simulink model "Torque_Vectoring_Controller_Boon"  (R2016a)
settings: Solver=ode45  StartTime=0.0  StopTime=inf  RelTol=1e-3
InitFcn:
  | clear_close
  | dataCar
  | optParam
  | structSensors
  | structSettings
  | structEstimPar
  | structAero
  | structVariables
  | readFuzzyFile
StartFcn:
  | clear_close
  | dataCar
  | optParam
  | structSensors
  | structSettings
  | structEstimPar
  | structAero
  | structVariables
  | readFuzzyFile
values from neighbouring files (symbols this model uses):
  mu = [0.05;0.05;0.05;0.05]    [frictionfrank.m]
undefined symbols (not defined in the file or in its folder): car, optPar, tire_radius
libraries: CarMaker4SL x42, simulink x11, fuzblock x1
(part 3 of 3)

== matlab function Torque_Vectoring_Controller_Boon/CarMaker/Controls/Control Systems/Traction Control ==
  data: sensors input; Torques output; settings input; estimPar input; torqueDistribution input; slipSet input; car parameter; TiTi2 output; error output
function [Torques, TiTi2, error] = Traction(sensors, settings, estimPar, torqueDistribution, slipSet, car)

error =[0 0 0 0]';
persistent errorInt; if isempty(errorInt); errorInt=[0 0 0 0]'; end
persistent errorD; if isempty(errorD); errorD=[0 0 0 0]'; end
persistent errorPrev; if isempty(errorPrev); errorPrev=[0 0 0 0]'; end

%persistent wi_prev; if isempty(wi_prev); wi_prev=[0 0 0 0]'; end
%persistent SR_expected; if isempty(SR_expected); SR_expected=zeros(4, 8); end
%persistent wvi_prev; if isempty(wvi_prev); wvi_prev=[0 0 0 0]'; end

persistent TiPrev; if isempty(TiPrev); TiPrev=[0 0 0 0]'; end

persistent errorInt2; if isempty(errorInt2); errorInt2=[0 0 0 0]'; end
persistent Ti; if isempty(Ti); Ti=[0 0 0 0]'; end
persistent Ti2; if isempty(Ti2); Ti2=[0 0 0 0]'; end


if settings.TC == 1

    slipRatioTarget = slipSet;
    dist = estimPar.Fzi/sum(estimPar.Fzi);
    
    Kp = 100*dist*10;
    Ki = 40*dist*1000;
    Kd = 0*dist/100;
    Kv = 70/100;
    Mu = 140;
    
    Kp2 = 20*dist/1000;
    Ki2 = 40*dist/1000;
    
    %normal non linear torque control
    error = slipRatioTarget - estimPar.slip;
    
    errorInt = errorInt + error*car.dt;
    errorInt = min(max(errorInt,-0.001*[1;1;1;1]),0.003*[1;1;1;1]);
    errorD = min(max(errorD*0.1 + 0.9*(error - errorPrev)/car.dt,-25),25);
    lambdaD = Kp.*error + Ki.*errorInt + Kd.*errorD;
    Ti = lambdaD*car.tireInertia*max(estimPar.v,0)^Kv/car.tireRadius + sign(torqueDistribution).*estimPar.Fzi*(Mu/100)*car.tireRadius;
    Ti = Ti / car.gearRatio;
    
    %optimum seeking
    dFds = dFdsCalculator(estimPar.Fxi,estimPar.slip);
    error2 = dFds - 0;
    errorInt2 = errorInt2 + error2*car.dt;
    errorInt2 = min(max(errorInt2,-500*[1;1;1;1]),500*[1;1;1;1]);
    lambdaD2 = Kp2.*error2 + Ki2.*errorInt2;
    Ti2 = lambdaD2*car.tireInertia*max(estimPar.v,0)^Kv/car.tireRadius + sign(torqueDistribution).*estimPar.Fzi*(car.TC_mu)*car.tireRadius;
    Ti2 = Ti2 / car.gearRatio;
    
%     for i=1:4
%         if abs(error(i)) < 0.05
%             Ti(i) = Ti2(i);
%         end
%     end
    
    if estimPar.v < 1/3.6
        %Ti = [80 80 180 180]';
        errorInt = [0 0 0 0]';
    end

    if sensors.throttle < 0.1
        errorInt = [0 0 0 0]';
    end
    
    lowerBoundary = TiPrev - 100/car.gearRatio;
    upperBoundary = TiPrev + 100/car.gearRatio;

    Ti = min(max(Ti,lowerBoundary),upperBoundary);
    
    TiPrev = Ti;
    errorPrev = error;
    
    Torques = Ti;
    for i=1:4
        if torqueDistribution(i) > 0
            Torques(i) = max(min(Torques(i),torqueDistribution(i)),0); 
        else
            Torques(i) = min(max(Torques(i),torqueDistribution(i)),0);
        end
    end
    
    
else
    Torques = torqueDistribution;
end

checkTorquemax = find((Torques > car.motor.Tmax)==1); %Limit torques to max torque
Torques(checkTorquemax)=car.motor.Tmax(checkTorquemax);



%wi_prev = sensors.wheelspeed;
%wvi_prev = sensors.wheelspeedi;

TiTi2 = [Ti;Ti2];

end

function [dFds] = dFdsCalculator(Fx,slipRatio)
N = 6;

persistent slipVector, if isempty(slipVector); slipVector = zeros(N,4); end
persistent FxVector, if isempty(FxVector); FxVector = zeros(N,4); end


FxVector(1,:) = Fx;
slipVector(1,:) = slipRatio;

dFds = [0;0;0;0];

for i=1:4
    p1 = polyfit(slipVector(:,i),FxVector(:,i),1);
    p2 = polyfit(FxVector(:,i),slipVector(:,i),1);
    
    rico1 = p1(1);
    rico2 = 1/p2(1);
    
    rico = sign(min(abs(rico1),abs(rico2)))*min(abs(rico1),abs(rico2));

    dFds(i) = max(min(rico,20000),-20000);
end

% shift list one
dummy = FxVector(1:N-1,:);
FxVector = [[0,0,0,0];dummy];
dummy = slipVector(1:N-1,:);
slipVector = [[0,0,0,0];dummy];

end

== matlab function Torque_Vectoring_Controller_Boon/CarMaker/Controls/Vehicle Estimated Parameters/Mu&Slip Estimator ==
  data: sensors input; mu output; settings input; slip output; v input; car parameter
function [mu,slip]= mu_slip(sensors, settings,v,car)
if isempty(v); v =0;end
yawRate = [0;0;sensors.yawRate];
dist = [car.lf car.lf -car.lr -car.lr;
    car.tw/2 -car.tw/2 car.tw/2 -car.tw/2;
    0 0 0 0];
wheelAngle = (sensors.wheelAngles(1)+sensors.wheelAngles(2))/2;

mu=[1.3;1.3;1.3;1.3];

omegaR = sensors.wheelspeed*car.tireRadius;
vWheel=zeros(4,1);
vWheel_m=zeros(3,4);

for i=1:4;
    v_sleep=cross(yawRate,dist(:,i));
    vWheel_m(:,i) = [v;0;0] + v_sleep;
    vWheel(i,1) = sqrt(vWheel_m(1,i)^2+vWheel_m(2,i)^2);
end



if sensors.ax > 0
    slip = (omegaR - vWheel)./omegaR;
elseif sensors.ax < 0
    slip = (omegaR - vWheel)./vWheel;
else
    slip = [0;0;0;0];
end
end

== matlab function Torque_Vectoring_Controller_Boon/CarMaker/Controls/Control Systems/Yaw Rate Control ==
  data: sensors input; Mz output; settings input; estimPar input; car parameter; error output; actions output; rref output
function [Mz,error,actions,rref]= yawRateControl(sensors, settings, estimPar, car)
%Function that controls the moment around the z-axis
%INPUTS:
%OUTPUT: Moment of the car around Z-axis [Nm]

Mz = 0;
Mz_temp = 0;
rref = estimPar.rref;
error = 0;


wheelAngle = (sensors.wheelAngles(1)+sensors.wheelAngles(2))/2;

%For analyzation
P_Action = 0;
I_Action = 0;
D_Action = 0;

steeringWheel_Action = 0;
yawRate_Action = 0;

persistent Mz_memory; if isempty(Mz_memory); Mz_memory = 0; end
persistent integral; if isempty(integral); integral = 0; end
persistent derivative; if isempty(derivative); derivative = 0; end
persistent prevError; if isempty(prevError); prevError = 0; end

%if settings.YRCMode == 1
error = estimPar.rref - sensors.yawRate;
integral = integral + error*car.dt;
integral = min(max(integral,-car.YRC.intLimit),car.YRC.intLimit);
derivative = (error - prevError)/car.dt;

Mz_temp = car.YRC.Kp*error + car.YRC.Ki*integral + car.YRC.Kd*derivative...
    +car.YRC.Ks*wheelAngle + car.YRC.Kr*estimPar.rref;
Mz_temp = max(min(Mz_temp,car.YRC.maxValue),-car.YRC.maxValue);
Mz_memory=Mz_memory+Mz_temp;

P_Action = car.YRC.Kp*error;
I_Action = car.YRC.Ki*integral;
D_Action = car.YRC.Kd*derivative;
steeringWheel_Action = car.YRC.Ks*wheelAngle;
yawRate_Action = car.YRC.Kr*estimPar.rref;

actions = [P_Action;I_Action;D_Action;steeringWheel_Action;yawRate_Action];
prevError = error;
%end


% if settings.YRCMode == 2
%     error = estimPar.rref - sensors.yawRate;
%     integral = integral + error*car.dt;
%     derivative = (error - prevError)/car.dt;
%
%     Mz_temp = car.YRC.Kp*error + car.YRC.Ki*integral + car.YRC.Kd*derivative...
%         +car.YRC.Ks*wheelAngle + car.YRC.Kr*estimPar.rref;
%     Mz_temp = max(min(Mz_temp,car.YRC.maxValue),-car.YRC.maxValue);
%
%     prevError = error;
% end





%YRC enabled
if settings.YRC ==1
    Mz = Mz_memory;
    %Mz = estimPar.rref;
    %YRC disabled
else
    Mz = 0;
end

if car.YRC.minV > estimPar.v
    Mz = 0; %if speed is too low, don't activate yaw rate control
    integral = 0;
    prevError = 0;
end



rref=estimPar.rref;

== matlab function Torque_Vectoring_Controller_Boon/CarMaker/Controls/Controller Settings/Controller Settings ==
  data: settings output Bus: settingBus; sensors input; variables output Bus: variableBus
function [settings,variables] = settingController(sensors)

%% Settings
velocityEstimation_Temp = 1;
YRCMode_Temp = 1;
torqueMode_Temp = 0;
YRC_Temp = 0;
TC_Temp = 0;
unlimitedFx_Temp = 0;

%if sensors.knob1 == 1
    YRC_Temp = 1;
%end

%if sensors.knob1 == 1
    torqueMode_Temp = 2; %Change distributor mode
%end

%if sensors.knob2 == 1
    YRCMode_Temp = 1;
    TC_Temp = 1;
    unlimitedFx_Temp = 0;
%end

%if sensors.knob2 == 2
    %YRCMode_Temp = 2;
%end

%% Variables
TD_percentage_Temp = 1;


%% Declaration Settings

settings.velocityEstimation = velocityEstimation_Temp;
settings.torqueMode = torqueMode_Temp;
settings.YRC = YRC_Temp;
settings.YRCMode = YRCMode_Temp;
settings.distributorMode = 0;

settings.Fsens = 100; %value between 0 and 100
% 100 --> Fdes is really important
% 0 --> Mdes is really important

settings.Fxsens = 1;

settings.TC = TC_Temp;
settings.unlimitedFx = unlimitedFx_Temp;

%% Declaration Variables
variables.TD_percentage = TD_percentage_Temp;

== matlab function Torque_Vectoring_Controller_Boon/CarMaker/Controls/Vehicle Estimated Parameters/Fz Estimator  ==
  data: sensors input; Fzi output; settings input; v input; car parameter; aero input
function Fzi = Fz_Estimator(sensors, settings, v,car, aero)
if isempty(v); v =0;end
%Dynamical loads 
%Without taking suspension into account


FFA = car.g*car.mass*car.lr/car.wb - (car.h/car.wb)*(car.mass*sensors.ax) - aero.FD*((car.h+aero.lever_FD(2))/car.wb) - aero.FL*((car.lr-aero.lever_FL(1))/car.wb); %dyn load Front Axle
FRA = car.g*car.mass*car.lf/car.wb + (car.h/car.wb)*(car.mass*sensors.ax) + aero.FD*((car.h+aero.lever_FD(2))/car.wb) - aero.FL*((car.lf+aero.lever_FL(1))/car.wb); %dyn load Rear Axle


FFL = FFA/2 - (car.h/(2*car.tw))*(car.mass*sensors.ay);
FFR = FFA/2 + (car.h/(2*car.tw))*(car.mass*sensors.ay);
FRL = FRA/2 - (car.h/(2*car.tw))*(car.mass*sensors.ay);
FRR = FRA/2 + (car.h/(2*car.tw))*(car.mass*sensors.ay);


Fzi = [FFL;FFR;FRL;FRR];

== matlab function Torque_Vectoring_Controller_Boon/CarMaker/Controls/Vehicle Estimated Parameters/Fx Estimator  ==
  data: sensors input; Fxi output; settings input; v input; car parameter; inertiaOut output; alpha output
function [Fxi,inertiaOut, alpha]= Fx_Estimator(sensors, settings, v, car)
%OPM: gearratio zit al verwerkt in sensors.torque (= wheelTorque)

persistent wheelspeedPrev; if isempty(wheelspeedPrev); wheelspeedPrev = [0 ;0 ;0 ;0]; end
persistent inertia; if isempty(inertia); inertia = car.tireInertia; end
if isempty(v); v =0;end
wheelspeed = sensors.wheelspeed;
alpha = (wheelspeed - wheelspeedPrev)/car.dt;

%wheelTorque = car.gearRatio*sensors.torque -(car.motor.Inertia*car.gearRatio^2 - car.tireInertia)*alpha;
%to be used if only motor torque is known (real scenario)

%Fxi_est = (wheelTorque - alpha*inertia)/car.tireRadius;
Fxi_est = (sensors.torque - alpha*inertia)/car.tireRadius;
%Fxi_est = (sensors.torque)/car.tireRadius;

Fx_tot = sensors.ax*car.mass + 0.5*car.rhoAir*v^2*car.Cd*car.AFront;
Fxi = Fxi_est;




wheelspeedPrev=wheelspeed;
inertiaOut = inertia;

== matlab function Torque_Vectoring_Controller_Boon/CarMaker/Controls/Vehicle Estimated Parameters/Velocity Estimator/Velocity Estimator 1 ==
  data: sensors input; v1 output; settings input; car parameter
function v1  = Velocity_Estimator1(sensors, settings,  car)

%x-axis forward
%y-axis left
%z-axis upwards

tw_dist = [car.tw/2; -car.tw/2; car.tw/2; -car.tw/2];    

omegaR = max(sensors.wheelspeed*car.tireRadius,0);

persistent v_last; if (isempty(v_last)); v_last = 0; end

%estimate vi
vi = omegaR - tw_dist.*sensors.yawRate;
vi = vi .* cos(sensors.wheelAngles); 

%Front/rear best speed estimation
ax=sensors.ax;
limitax = 10;

vl = vi([1 3]);
vr = vi([2 4]);

if (ax > limitax)
   vsetl=min(vl);
   vsetr=min(vr);
elseif (ax < -limitax)
   vsetl=max(vl);
   vsetr=max(vr);
else
   vsetl=(min(vl)*(limitax + ax) + max(vl)*(limitax - ax))/(2*limitax);
   vsetr=(min(vr)*(limitax + ax) + max(vr)*(limitax - ax))/(2*limitax);
end
    
%left/right best speed estimation
ay=sensors.ay;
limitay = 20;

if (ay > limitay)
   v_est = vsetr;
elseif (ay < -limitay)
   v_est = vsetl;
else
   v_est = (vsetr*(ay + limitay) + vsetl*(limitay-ay))/(2*limitay);
end

v1=v_est;
%v=mean(omegaR);

== matlab function Torque_Vectoring_Controller_Boon/CarMaker/Controls/Control Systems/Distributor/MATLAB Function ==
  data: sensors input; torqueDistribution output; settings input; estimPar input; car parameter; variables input; Mz input; slipSet output; Fdes output; sumFx output; Fxmax output; Fxmaxsum output; Fx output
function [torqueDistribution, slipSet,Fdes,sumFx,Fxmax,Fxmaxsum, Fx]= TorqueDistributor(sensors,settings, estimPar, car, variables, Mz)
%,Fdes,sumFx,Fxmax,Fxmaxsum

torqueDistribution = [0;0;0;0];
slipSet = [0;0;0;0];

Fdes=0;
sumFx=0;
Fxmax=[0;0;0;0];
Fxmaxsum=0;
Fx=[0;0;0;0];
if settings.torqueMode == 1
    
    dT =  0.25*Mz/(car.tw*0.5)*car.tireRadius;
    torqueDistribution = car.motor.Tmax*variables.TD_percentage*sensors.throttle;
    torqueDistribution = torqueDistribution + [-1; 1; -1; 1]*dT;
    
    for i=1:4
        if torqueDistribution(i) > 0
            slipSet(i) = car.TC.slipSetAcc;
        else
            slipSet(i) = car.TC.slipSetBrake;
        end
    end
    
    
end



%Test torque mode: only Fx, no steeringAngle

if settings.torqueMode == 2
    
    %Fdes = 11*4* min(car.motor.Tmax)*variables.TD_percentage*sensors.throttle/car.tireRadius;
    %if sensors.throttle > 0
    Fdes = sum(car.motor.Tmax)*variables.TD_percentage*sensors.throttle/car.tireRadius; % *4 because four motors
    Fdes = Fdes*car.gearRatio;
    
    if sensors.brake > 0
        Fdes = -sum(car.motor.Tmax)*variables.TD_percentage*sensors.brake/car.tireRadius;
        Fdes = Fdes*car.gearRatio;
    end
    %Fdes= 5000;
    
    %end
    %     Fdes = Fdes*1;
    %     Fdes = 800;
    
    %     Fdes = sensors.throttle*mean(estimPar.mu)*(car.mass*car.g + 0.5*car.rhoAir*estimPar.v*estimPar.v*car.Cl*car.AFront );
    %     Fdes = Fdes;
    
    
    Fxmax = [0;0;0;0];
    %minForce = 2*car.Cd*car.AFront*0.5*car.rhoAir*estimPar.v*estimPar.v*0.25; %2* of niet? en met Cd?
    minForce = 0;
    %FyReduceFactor = 0.1;
    %Fxmax = (max((estimPar.mu .* estimPar.Fzi).^2-FyReduceFactor*estimPar.Fyi.^2,0).^0.5); %Kamm's circle
    
    
    
    Fxmax = estimPar.mu.*estimPar.Fzi;
    
    Fxmax = max(Fxmax,minForce);
    
    FxmaxMax = car.gearRatio*car.motor.Tmax/car.tireRadius; %make sure the max torque of the motor isn't surpassed
    checkFxmax = find((Fxmax > FxmaxMax)==1);
    Fxmax(checkFxmax)=FxmaxMax(checkFxmax);
    
    if settings.unlimitedFx == 1  %Surpass the tire grip limits in case if the driver feels to restricted with this.
        Fxmax = FxmaxMax;
    end
    
    Fxmaxsum = sum(Fxmax);
    Fxmin = -Fxmax;
    
    Fx = [0;0;0;0];
    
    
    Fx = Distributor(settings, car, Mz, Fdes, Fxmax, Fxmin);
    
    torqueDistribution = car.tireRadius*Fx; %torque of motor, NOT of wheels (as IPG expects this as input)
    
    for i=1:4
        if torqueDistribution(i) > 0
            slipSet(i) = car.TC.slipSetAcc;
        else
            slipSet(i) = car.TC.slipSetBrake;
        end
    end
    
    sumFx = sum(Fx);
end


end

== matlab function Torque_Vectoring_Controller_Boon/CarMaker/Controls/Control Systems/Slip Rate Control ==
  data: sensors input; y output; settings input; estimPar input
function y = fcn(sensors, settings, estimPar)

y = u;

== matlab function Torque_Vectoring_Controller_Boon/CarMaker/Controls/Vehicle Estimated Parameters/Velocity Estimator/Velocity_Estimator4 ==
  data: sensors input; v4 output; settings input; Fyi input; car parameter
function v4  = Velocity_Estimator4(sensors, settings,Fyi,  car)

% Based on "Vehicle velocity estimation using effective inertia for an in-wheel
% elecric vehicle"

SumLongitudinalForce=0;




persistent wheelspeedPrev; if isempty(wheelspeedPrev); wheelspeedPrev = [0 ;0 ;0 ;0]; end
persistent vPrev; if isempty(vPrev); vPrev = 0; end
persistent v4dot; if isempty(v4dot); v4dot = 0; end
wheelspeed = sensors.wheelspeed;

alpha = (wheelspeed - wheelspeedPrev)/car.dt;

Fresist = 0.5*car.Cd*car.AFront*car.rhoAir*vPrev^2; % moet nauwkeuriger


SumLongitudinalForce = sum(sensors.torque-alpha*car.tireInertia)/car.tireRadius...
    - Fresist;
Meff = SumLongitudinalForce/sensors.ax; %effective inertia / virtual mass


v4dot = (-(Fyi(1)*sin(sensors.wheelAngles(1))+Fyi(2)*sin(sensors.wheelAngles(2)))...
    + SumLongitudinalForce) / Meff;




v4 = vPrev + v4dot*car.dt;

vPrev = v4;




end

== matlab function Torque_Vectoring_Controller_Boon/CarMaker/Controls/Vehicle Estimated Parameters/Fy Estimator  ==
  data: sensors input; Fyi output; settings input; Fzi input; Fxi input; car parameter; optPar parameter
function Fyi = Fy_Estimator(sensors, settings, Fzi, Fxi, car,optPar)

Fyi=[0;0;0;0];
persistent yawRatePrev; if isempty(yawRatePrev); yawRatePrev = sensors.yawRate; end
persistent M_Fx; if isempty(M_Fx); M_Fx = 0; end
persistent M_Fy; if isempty(M_Fy); M_Fy = 0; end
persistent FyRear; if isempty(FyRear); FyRear = 0; end
persistent FzRatioFront; if isempty(FzRatioFront);FzRatioFront = 0; end
persistent FzRatioRear; if isempty(FzRatioRear); FzRatioRear = 0; end
persistent FyFront; if isempty(FyFront); FyFront = 0; end
persistent Fy_FL; if isempty(Fy_FL); Fy_FL = 0; end

yawAcc = (sensors.yawRate - yawRatePrev) * car.fECU;

wheelAngle = (sensors.wheelAngles(1)+sensors.wheelAngles(2))/2;

%Calculate contributions to the moment from lateral forces through the
%total yaw moment and moment of the longitudinal forces.
M_YawTot = car.yawInertia*yawAcc;
M_Fx = (car.tw/2)*cos(wheelAngle)*(Fxi(1)-Fxi(2))...
    +car.lf*sin(wheelAngle)*(Fxi(1)+Fxi(2))...
    +(car.tw/2)*(Fxi(3)-Fxi(4));
M_Fy = M_YawTot - M_Fx;

%Distribution of lateral force on front and rear axle
%NOTE %sin(steerinAngle) deel wordt momenteel verwaarloosd
%     %--> FyFR - FyFL =~ 0
Fy = car.mass*sensors.ay;
FyRear = (cos(wheelAngle)*car.lf*Fy - M_Fy)/...
    (cos(wheelAngle)*car.lf+car.lr);
FyFront = Fy - FyRear;

%Distribution of lateral force on left and right tire by using the normal
%force distribution.

%Use of a scale factor 

FzRatioFront = [Fzi(1); Fzi(2)]./sum(Fzi(1:2));
FzRatioRear = [Fzi(3); Fzi(4)]./sum(Fzi(3:4));



FyFrontDiff = (FzRatioFront(1) - FzRatioFront(2))*optPar.scaleFactorFy/2;
Fy_FL = FyFront/2 + FyFrontDiff* FyFront;
Fy_FR = FyFront/2 - FyFrontDiff* FyFront;
FyRearDiff = (FzRatioRear(1) - FzRatioRear(2))*optPar.scaleFactorFy/2;
Fy_RL = FyRear/2 + FyRearDiff* FyRear;
Fy_RR = FyRear/2 - FyRearDiff* FyRear;
    
Fyi=[Fy_FL;Fy_FR;Fy_RL;Fy_RR];

yawRatePrev=sensors.yawRate;

== matlab function Torque_Vectoring_Controller_Boon/CarMaker/IPG Feedback/Subsystem/MATLAB Function ==
  data: Wheelspeed_Max input; T_mot output; Wheelspeed_Sens input; Treq input
function T_mot = SpeedLimit(Wheelspeed_Max,Wheelspeed_Sens,Treq)
%Speed limiter for IPG Carmaker
if Wheelspeed_Sens>= Wheelspeed_Max
    T_mot=0;
else
    T_mot=Treq;
end

== matlab function Torque_Vectoring_Controller_Boon/CarMaker/Controls/Vehicle Estimated Parameters/Aerodynamic forces ==
  data: sensors input; aero output Bus: aeroBus; settings input; v input; car parameter
function aero = aerodynamics(sensors, settings, v, car)

% === from dataCar.m ===
% car.Cl = 3.84;      %[-]   %Lift coefficient
% car.Cd = 1.44;      %[-]   %Drag coefficient
% car.AFront = 1.3;   %[m^2] %Frontal area
% car.rhoAir = 1.225; %[kg/m^3] %air density

aero.FD = 0.5*car.Cd*car.AFront*car.rhoAir*v^2; %drag force, pointing rearward [N]
aero.FL = 0.5*car.Cl*car.AFront*car.rhoAir*v^2; %lift force, pointing upward [N]
aero.lever_FD = [-0.1;0.1]; %distance from the COG to the point of application of the drag [m]
aero.lever_FL = [-0.1;0.1]; %distance from the COG to the point of application of the lift [m]

== matlab function Torque_Vectoring_Controller_Boon/CarMaker/Controls/Vehicle Estimated Parameters/Estim Par ==
  data: v input; estimPar output Bus: estimParBus; Fzi input; Fxi input; Fyi input; rref input; mu input; slip input
function estimPar = fcn(v,Fzi,Fxi,Fyi,rref,mu,slip)

estimPar.v=v;
estimPar.Fzi=Fzi;
estimPar.Fxi=Fxi;
estimPar.Fyi=Fyi;
estimPar.rref=rref;
estimPar.mu=mu;
estimPar.slip=slip;

== matlab function Torque_Vectoring_Controller_Boon/CarMaker/Controls/Vehicle Estimated Parameters/Velocity Estimator/Velicity Estimator 2 ==
  data: sensors input; v2 output; settings input; car parameter; vCOG output
function [v2,vCOG] = Velocity_Estimator1(sensors, settings,  car)

vycog = 0;
dist = [car.lf car.lf -car.lr -car.lr;
  car.tw/2 -car.tw/2 car.tw/2 -car.tw/2;
  0 0 0 0];
wheelAngle = (sensors.wheelAngles(1)+sensors.wheelAngles(2))/2;

%tw_dist = [-car.tw/2 car.tw/2 -car.tw/2 car.tw/2];
      

% Note: axis systems X,Y,Z in car frame, x,y,z in wheel frame.
%X:forward
%Y:left
%Z:up


RxyzXYZ=[cos(wheelAngle) sin(wheelAngle) 0;
   -sin(wheelAngle) cos(wheelAngle) 0;
   0 0 1];
omega = [0 0 0 0 ;
   sensors.wheelspeed(1) sensors.wheelspeed(2) sensors.wheelspeed(3) sensors.wheelspeed(4)
   ;0 0 0 0];
radius = [0;0;-car.tireRadius];
yawRate = [0;0;sensors.yawRate];

% wheelspeed = [sensors.wheelspeed(1) sensors.wheelspeed(2) sensors.wheelspeed(3) sensors.wheelspeed(4)];
% steeringAngle = [wheelAngle;wheelAngle;0;0];
% omegaR = [sensors.wheelspeed(1); sensors.wheelspeed(2); sensors.wheelspeed(3); sensors.wheelspeed(4)].*car.tireRadius;


% persistent vCOG_m
% if isempty(vCOG_m); vCOG_m = zeros(3,4); end

% persistent vxCOG
% if isempty(vxCOG); vxCOG = zeros(4,1); end
vCOG_m = zeros(3,4);
vCOG = zeros(4,1);

%vxCOG_m = zeros(4,1);


%Can be faster without the matrices
%Slip can be taken into account by v_wheel(now=0,changing it to velocity with slip) =
%RxyzXYZ*cross(wheelspeed,tireRadius)+cross(yawRate,dist)+vXYZ
 
for i=1:4
    vCOG_m(:,i) = -(RxyzXYZ*cross(omega(:,i),radius)+cross(yawRate,dist(:,i)));  %%SteeringAngle is not yet changed for the rear wheels w
    vCOG(i,1) = sqrt(vCOG_m(1,i)^2+vCOG_m(2,i)^2);
    %vxCOG_m(i,1)=vCOG_m(1,i);
    %vxCOG(i,1)=-(cos(steeringAngle(i))*(car.tireRadius*wheelspeed(i))-sensors.yawRate*tw_dist(i));
end

% Select/average based on wheel speed
axtol = 2; % Tolerance to detect acceleration / deceleration [m/s2]
if sensors.ax > axtol
    vEst_wheels = min(vCOG);    %lowest wheelspeed to take possible slip into account
elseif sensors.ax < -axtol
    vEst_wheels = max(vCOG);    %highest wheelspeed to take possible wheel lock into account
else
    vEst_wheels = median(vCOG); % Note: median is less sensitive to outliers
end




v2= vEst_wheels;

== matlab function Torque_Vectoring_Controller_Boon/CarMaker/Controls/Vehicle Estimated Parameters/Velocity Estimator/Velocity_Estimator3 ==
  data: sensors input; v3 output; settings input; car parameter; v input
function v3  = Velocity_Estimator3(sensors, settings,  car, v)

persistent vActual; if isempty(vActual); vActual = 0; end


%IMPORTANT: change car.fECU and car.dt when changing operating speed in Simulink

v3 = vActual + sensors.ax * car.dt;

vActual = v;

== matlab function Torque_Vectoring_Controller_Boon/CarMaker/IPG Feedback/Subsystem/MATLAB Function1 ==
  data: Wheelspeed_Max input; T_mot output; Wheelspeed_Sens input; Treq input
function T_mot = SpeedLimit(Wheelspeed_Max,Wheelspeed_Sens,Treq)
%Speed limiter for IPG Carmaker
if Wheelspeed_Sens>= Wheelspeed_Max
    T_mot=0;
else
    T_mot=Treq;
end

== matlab function Torque_Vectoring_Controller_Boon/CarMaker/IPG Feedback/Subsystem/MATLAB Function2 ==
  data: Wheelspeed_Max input; T_mot output; Wheelspeed_Sens input; Treq input
function T_mot = SpeedLimit(Wheelspeed_Max,Wheelspeed_Sens,Treq)
%Speed limiter for IPG Carmaker
if Wheelspeed_Sens>= Wheelspeed_Max
    T_mot=0;
else
    T_mot=Treq;
end

== matlab function Torque_Vectoring_Controller_Boon/CarMaker/IPG Feedback/Subsystem/MATLAB Function3 ==
  data: Wheelspeed_Max input; T_mot output; Wheelspeed_Sens input; Treq input
function T_mot = SpeedLimit(Wheelspeed_Max,Wheelspeed_Sens,Treq)
%Speed limiter for IPG Carmaker
if Wheelspeed_Sens>= Wheelspeed_Max
    T_mot=0;
else
    T_mot=Treq;
end

== matlab function Torque_Vectoring_Controller_Boon/CarMaker/Controls/Vehicle Estimated Parameters/Velocity Estimator/MATLAB Function ==
  data: v1 input; v2 input; v output; v3 input; v4 input; vKalman input; vFuzzy input
function v = fcn(v1,v2,v3,v4,vKalman,vFuzzy)
%#codegen

v = vFuzzy;

== matlab function Torque_Vectoring_Controller_Boon/CarMaker/Controls/Vehicle Estimated Parameters/Velocity Estimator/Kalman Velocity ==
  data: sensors input; settings input; v2 input; vKalman output; v4 input; car parameter
function vKalman = Velocity_EstimatorKalman(sensors,settings,v2,v4,car)


% Keep track of the estimated velocity
persistent vEst; if isempty(vEst); vEst = 0; end;
persistent PEst; if isempty(PEst); PEst = 0; end;

% Model
A = 1; B = car.dt;
H = [1;1];
Q = car.kalmanVelocity.Q;
R = car.kalmanVelocity.R;

% Measurements
y = [v2; v4];

% if settings.velocityEstimation == 0 || settings.velocityEstimation == 1 || vEst < car.speed.velTreshold || sensors.vboxX < car.speed.velTreshold
%     %vbox disabled
%     H(1) = 0;
% end



% === Time update ===
vEst = A*vEst + B*sensors.ax;
PEst = A*PEst*A' + Q;

% === Measurement update ===
K = PEst*H'/(H*PEst*H'+R);
vEst = vEst + K*(y-H*vEst);
PEst = (1-K*H)*PEst;
% Output
vest_out = vEst;

%sensors_out = sensors;
%sensors_out.vx = vest_out;
vKalman = vest_out;

== matlab function Torque_Vectoring_Controller_Boon/CarMaker/Controls/Vehicle Estimated Parameters/Velocity Estimator/Fuzzy Velocity/FuzzyVelicityGenerator ==
  data: k1 input; vFuzzy output; k2 input; k3 input; k4 input; k5 input; sensors input; settings input; car parameter
function vFuzzy = fuzzyVelocityGenerator(k1,k2,k3,k4,k5,sensors,settings,car)

persistent vFuzzyPrev; if isempty(vFuzzyPrev); vFuzzyPrev = 0; end

beta=0;


vRFL_COG = (sensors.wheelspeed(1)*car.tireRadius...
    + sensors.yawRate*(car.tw/2-car.lf*beta))...
    *cos(sensors.wheelAngles(1)-beta);
vRFR_COG = (sensors.wheelspeed(2)*car.tireRadius...
    - sensors.yawRate*(car.tw/2+car.lf*beta))...
    *cos(sensors.wheelAngles(2)-beta);
vRRL_COG = (sensors.wheelspeed(3)*car.tireRadius...
    + sensors.yawRate*(car.tw/2+car.lr*beta))...
    *cos(beta);
vRRR_COG = (sensors.wheelspeed(4)*car.tireRadius...
    - sensors.yawRate*(car.tw/2-car.lr*beta))...
    *cos(beta);
vR_COG=[vRFL_COG;vRFR_COG;vRRL_COG;vRRR_COG];

vFuzzy = (sum([k1;k2;k3;k4].*vR_COG)+k5*(vFuzzyPrev+car.dt*sensors.ax))...
    /(k1+k2+k3+k4+k5);

vFuzzyPrev = vFuzzy;

== matlab function Torque_Vectoring_Controller_Boon/CarMaker/Controls/Vehicle Estimated Parameters/Velocity Estimator/Fuzzy Velocity/fuzzyParam ==
  data: sensors input; deltaVFL output; settings input; vFuzzyPrev input; deltaVFR output; deltaVRL output; deltaVRR output; maxDeltaV output; car parameter
function [deltaVFL,deltaVFR,deltaVRL,deltaVRR,maxDeltaV]= fuzzyParam(sensors, settings,vFuzzyPrev,car)
beta=0;
vRFL_COG = (sensors.wheelspeed(1)*car.tireRadius...
    + sensors.yawRate*(car.tw/2-car.lf*beta))...
    *cos(sensors.wheelAngles(1)-beta);
vRFR_COG = (sensors.wheelspeed(2)*car.tireRadius...
    - sensors.yawRate*(car.tw/2+car.lf*beta))...
    *cos(sensors.wheelAngles(2)-beta);
vRRL_COG = (sensors.wheelspeed(3)*car.tireRadius...
    + sensors.yawRate*(car.tw/2+car.lr*beta))...
    *cos(beta);
vRRR_COG = (sensors.wheelspeed(4)*car.tireRadius...
    - sensors.yawRate*(car.tw/2-car.lr*beta))...
    *cos(beta);
vR_COG=[vRFL_COG;vRFR_COG;vRRL_COG;vRRR_COG];

deltaVFL = vRFL_COG-vFuzzyPrev;
deltaVFR = vRFR_COG-vFuzzyPrev;
deltaVRL = vRRL_COG-vFuzzyPrev;
deltaVRR = vRRR_COG-vFuzzyPrev;

maxDeltaV = abs(vFuzzyPrev-max(vR_COG))+abs(vFuzzyPrev-min(vR_COG));

== matlab function Torque_Vectoring_Controller_Boon/CarMaker/Controls/Vehicle Estimated Parameters/Yaw Rate Reference ==
  data: sensors input; rref output; settings input; v input; car parameter
function rref = yawRateRef(sensors, settings, v, car)
if isempty(v); v =0;end
%Ackermann
wheelAngle = (sensors.wheelAngles(1)+sensors.wheelAngles(2))/2;
rref = wheelAngle*v/car.wb;




% 
% des_yaw_rate = vx*steering_angle / ...
%     (L_f + L_r + ...
%     m_chassis*vx^2*(L_r*(C_x_alpha_RL+C_x_alpha_RR)-L_f*(C_x_alpha_FL+C_x_alpha_FR))/...
%     ((C_x_alpha_RL+C_x_alpha_RR)*(C_x_alpha_FL+C_x_alpha_FR)*L));

== matlab function Torque_Vectoring_Controller_Boon/CarMaker/Vehicle Sensors/Sensors ==
  data: ax input; sensors output Bus: sensorBus size=1; ay input; wheelspeed_FL input; wheelspeed_FR input; wheelspeed_RL input; wheelspeed_RR input; yawRate input; steeringAngle input; steerAngleFL input; steerAngleFR input; throttle input; brake input; torqueFL input; torqueFR input; torqueRL input; torqueRR input; ax_error input; ay_error input; yawRate_error input; knob1 input; knob2 input
function sensors = sensors(ax,ay,wheelspeed_FL,wheelspeed_FR,wheelspeed_RL,wheelspeed_RR,yawRate,steeringAngle,steerAngleFL,steerAngleFR, throttle,brake,torqueFL,torqueFR,torqueRL,torqueRR,ax_error,ay_error,yawRate_error,knob1,knob2)

sensors.ax = ax;
sensors.ay = ay;
sensors.wheelspeed = [wheelspeed_FL;wheelspeed_FR;wheelspeed_RL;wheelspeed_RR];
sensors.yawRate = yawRate;
sensors.steerAngle = steeringAngle;
sensors.wheelAngles = [steerAngleFL;steerAngleFR;0;0];
sensors.throttle = throttle;
sensors.brake= brake;
sensors.torque = [torqueFL;torqueFR;torqueRL;torqueRR];
sensors.ax_error = ax_error;
sensors.ay_error = ay_error;
sensors.yawRate_error = yawRate_error;
sensors.knob1 = knob1;
sensors.knob2 = knob2;
